simulink model "WashingMc_Stateflow"  (R2020a)
settings: Solver=VariableStepAuto  StartTime=0.0  StopTime=15  RelTol=1e-3
undefined symbols (not defined in the file or in its folder): sigbuilder_block
settings Model: Creator=user  LastModifiedBy=user

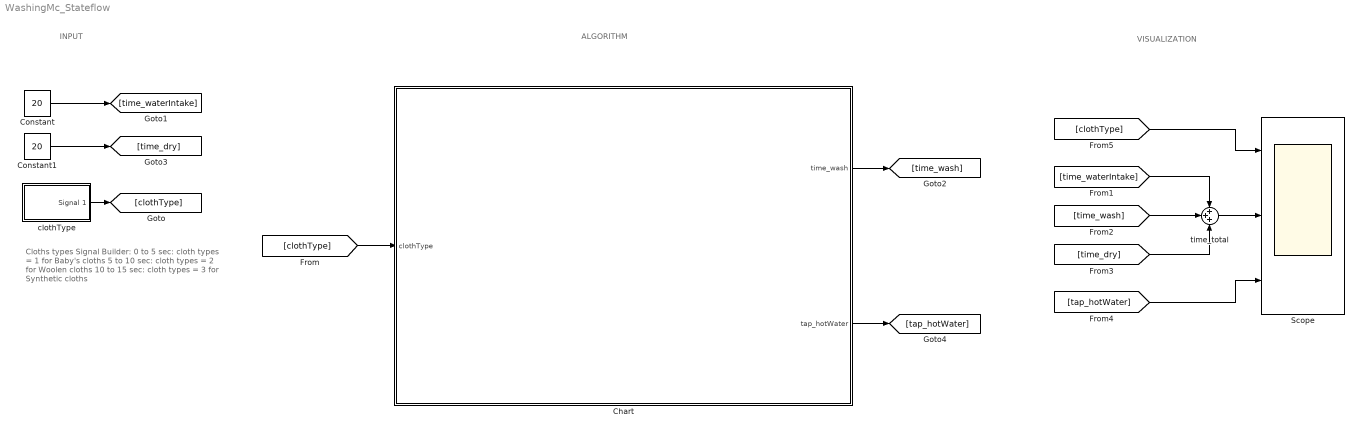
== system WashingMc_Stateflow ==
  note: Cloths types Signal Builder:
      | 0 to 5 sec: cloth types = 1 for Baby's cloths
      | 5 to 10 sec: cloth types = 2 for Woolen cloths
      | 10 to 15 sec: cloth types = 3 for Synthetic cloths
  note: VISUALIZATION
  note: ALGORITHM
  note: INPUT
  Chart : Stateflow chart  TreatAsAtomicUnit=on
  Constant : Constant  Value=20
  Constant1 : Constant  Value=20
  Scope : Scope  NumInputPorts=3
  clothType : Subsystem  Tag=STV Subsys  LoadFcn=sigbuilder_block('load',[437.6 199.2 550.4 400 ]);  StartFcn=sigbuilder_block('start');  StopFcn=sigbuilder_block('stop');  ClipboardFcn=sigbuilder_block('clipboard');  mask(Sigbuilder block){tuvar=[0:10]}
      mask help: Simulink:masks:SigbuilderBlock_MD
      mask init:
      | if ~strcmp(get_param(bdroot(gcbh),'SimulationStatus'),'stopped') tuvar = sigbuilder_block('maskInit'); end
      settings: CopyFcn=sigbuilder_block('copy');  DeleteFcn=sigbuilder_block('delete');  ModelCloseFcn=sigbuilder_block('modelClose');  PreSaveFcn=sigbuilder_block('preSave');  PauseFcn=sigbuilder_block('pause');  ContinueFcn=sigbuilder_block('continue');  NameChangeFcn=sigbuilder_block('namechange');  OpenFcn=sigbuilder_block('open',[437.6 199.2 550.4 400 ]);  CloseFcn=sigbuilder_block('close');
      mask Display: plot(0, 0, 100, 100,[2, 2, 32, 32, 2], [68, 8, 8, 68, 68],[32, 2], [38, 38], [32, 19, 2],[53, 60, 44], [32, 17, 17, 2],[16, 16, 31, 31]);txt = getActiveGroup(gcbh);text(2, 100, txt,'verticalAlignment', 'top');
  time_total : Sum  Inputs=+++
  wires:
  Constant/1 -> [time_waterIntake]
  Constant1/1 -> [time_dry]
  clothType/1(Signal 1) -> [clothType]
  [clothType] -> Chart/1(clothType)
  Chart/1(time_wash) -> [time_wash]
  Chart/2(tap_hotWater) -> [tap_hotWater]
  [time_wash] -> time_total/2
  [time_waterIntake] -> time_total/1
  [time_dry] -> time_total/3
  time_total/1 -> Scope/2
  [tap_hotWater] -> Scope/3
  [clothType] -> Scope/1

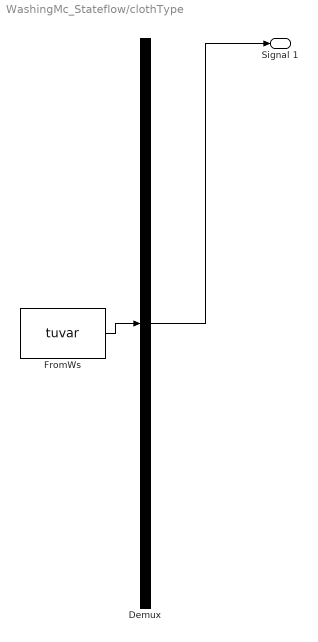
== system WashingMc_Stateflow/clothType ==
  Demux : Demux  Tag=STV Demux  Outputs=1
      settings: DisplayOption=none
  FromWs : FromWorkspace  Tag=STV FromWs  VariableName=tuvar
      SigBuilderData=|
      | common.afterFinalStr = 'Extrapolate'
      | common.sampleTime = 0
      | dataSet.timeRange = [0 15]
      | dataSet.name = 'Group 1'
      | sbobj.Groups.Name = 'Group 1'
      | sbobj.Groups.Signals.Name = 'Signal 1'
      | sbobj.Groups.Signals.XData = [0 5 5 10 10 15]
      | sbobj.Groups.Signals.YData = [1 1 2 2 3 3]
      | sbobj.Groups.TimeRange = [0 15]
  Signal 1 : Outport  Tag=STV Outport
  wires:
  Demux/1 -> Signal 1/1
  FromWs/1 -> Demux/1

== stateflow chart WashingMc_Stateflow/Chart ==
  state BABY_CLOTHTYPE_1
    entry:
    time_wash = 10;
    tap_hotWater = 1;
  state WOOLEN_CLOTHTYPE_2
    entry:
    time_wash = 15;
    tap_hotWater = 0;
  state SYNTHETIC_CLOTHTYPE_3
    entry:
    time_wash = 20;
    tap_hotWater = 0;
  (default) -> BABY_CLOTHTYPE_1
  BABY_CLOTHTYPE_1 -> WOOLEN_CLOTHTYPE_2 [order 1] : [clothType == 2]
  WOOLEN_CLOTHTYPE_2 -> BABY_CLOTHTYPE_1 [order 1] : [clothType == 1]
  BABY_CLOTHTYPE_1 -> (junction 10) [order 2]
  (junction 9) -> BABY_CLOTHTYPE_1 : [clothType == 1]
  WOOLEN_CLOTHTYPE_2 -> (junction 12) [order 2] : [clothType == 3]
  (junction 11) -> WOOLEN_CLOTHTYPE_2 : [clothType == 2]
  (junction 12) -> SYNTHETIC_CLOTHTYPE_3
  SYNTHETIC_CLOTHTYPE_3 -> (junction 9) [order 1]
  (junction 10) -> SYNTHETIC_CLOTHTYPE_3 : [clothType == 3]
  SYNTHETIC_CLOTHTYPE_3 -> (junction 11) [order 2]
  data: clothType input; time_wash output; tap_hotWater output
